simulink model "MMAE_beh_id_and_HighD"  (R2019b)
settings: Solver=FixedStepAuto  StartTime=0.0  StopTime=12  FixedStep=Ts_bp  RelTol=1e-3
values from neighbouring files (symbols this model uses):
  Ts = 0.1    [KinematicBicycleModel.m]    (also in LeftLaneChangeSinusoidalMotionModel.m; LinearizedBicycleModel.m; SimplifiedKinematicBicycleModel.m; amm_rel_test.m)
  Ts_bp = 0.01    [laneChangeSinusoidalFcn.m]    (also in laneChangeSinusoidalJacobianFcn.m; leftLaneChangeParametricFcn.m; leftLaneChangeParametricWithAccFcn.m; leftLaneChangeRelativeFcn.m = 0.1)
  vx = X(2)    [cv_model_fun.m]
  vy = X(4)    [cv_model_fun.m]
  x = X(1)    [KinematicBicycleModel.m]    (also in SimplifiedKinematicBicycleModel.m; behavior_model.m = 0:0.01:20; cca_model_fun.m; ctra_model_fun.m)
  y = X(2)    [KinematicBicycleModel.m]    (also in SimplifiedKinematicBicycleModel.m; behavior_model.m = [distances velocities]; cca_model_fun.m; ctra_model_fun.m)
undefined symbols (not defined in the file or in its folder): ax, P_init, rel_x, sigbuilder_block
libraries: simulink x8, dspswit3 x2, dspstat3 x2
settings Model: Creator=jasprit  LastModifiedBy=jasprit
settings DataIOCC: ReturnWorkspaceOutputs=off
settings DebuggingCC: UnderSpecifiedDimensionMsg=warning  ArithmeticOperatorsInVariantConditions=warning
settings SFSimCC: SimUseLocalCustomCode=off  CustomCodeUndefinedFunction=UseInterfaceOnly
settings RTWCC: RTWUseLocalCustomCode=off

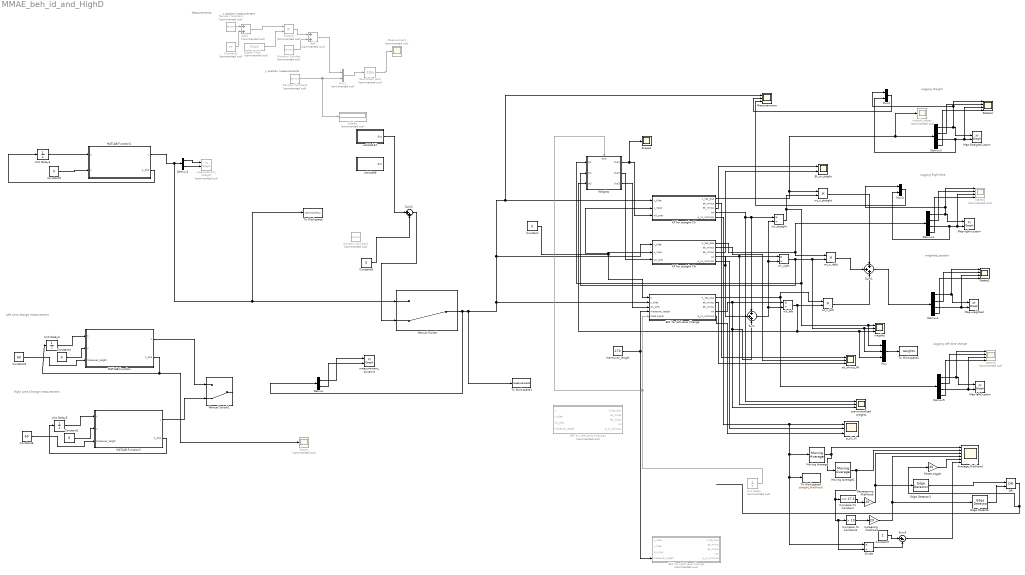
== system MMAE_beh_id_and_HighD ==
  note: Left Lane change measurement
  note: Right Lane Change measurement
  note: Logging Left lane change
  note: Logging straight
  note: Logging Right lane
  note: y position measurements
  note: x position measurement
  note: Measurements
  note: weighted_position
  Add : Sum  Commented=on
  Add1 : Sum  Commented=on
  Average_likelihood : Scope  NumInputPorts=6
  Compare To Constant : simulink/Logic and Bit Operations/Compare To Constant  relop=<=  const=27.5  OutDataTypeStr=boolean
  Compare To Constant1 : simulink/Logic and Bit Operations/Compare To Constant  relop=>  const=10  OutDataTypeStr=boolean
  Constant : Constant  Value=0
  Constant1 : Constant  Value=0  SampleTime=-1
  Constant2 : Constant  Commented=on  Value=vx  SampleTime=Ts
  Constant3 : Constant  Value=60
  Constant4 : Constant  Value=0  SampleTime=-1
  Constant5 : Constant  Value=0  SampleTime=-1
  Constant6 : Constant  Value=60
  Constant7 : Constant
  Constant8 : Constant  Value=0
  Decreasomg likelihood : Gain  Gain=20
  Demux : Demux  Outputs=2
  Demux{1,3..5} (4 alike) : Demux
  Demux2 : Demux  Outputs=2
  Digital Clock : DigitalClock  Commented=on  SampleTime=Ts
  Display : Display  Commented=on
  Divide : Product  Inputs=*/
  EKF for Left Lane Change1 : Subsystem  Commented=on
  EKF for left Lane Change : Subsystem  TreatAsAtomicUnit=on
  EKF for right Lane Change : Subsystem  Commented=on
  Edge Detector : dspswit3/Edge Detector
      settings: SourceProductName=DSP System Toolbox  SourceProductBaseCode=DS
  Edge Detector1 : dspswit3/Edge Detector
      settings: SourceProductName=DSP System Toolbox  SourceProductBaseCode=DS
  Ek_m_stright : Scope  NumInputPorts=2
  Increasing likelihood : Gain  Gain=20
  KF for straight CA : Subsystem
  KF for straight CV : Subsystem
  MATLAB Function : MATLAB Function  TreatAsAtomicUnit=on
  MATLAB Function1 : MATLAB Function  TreatAsAtomicUnit=on
  MATLAB Function2 : MATLAB Function  TreatAsAtomicUnit=on
  Manual Switch : ManualSwitch  CurrentSetting=0
  Manual Switch1 : ManualSwitch  CurrentSetting=0
  Map-StraightCustom : simulink/Sinks/XY Graph  xmin=-1  xmax=200  ymin=-20  ymax=20  st=-1
  Map-leftCustom : simulink/Sinks/XY Graph  xmin=-1  xmax=300  ymin=-5  ymax=5  st=-1
  Map-right-custom : simulink/Sinks/XY Graph  xmin=-1  xmax=300  ymin=-5  ymax=5  st=-1
  Map-weighted : simulink/Sinks/XY Graph  xmin=-1  xmax=300  ymin=-5  ymax=5  st=-1
  "Measurement " : Scope  Commented=on
  Measurements : Scope  NumInputPorts=3
  Moving Average : dspstat3/Moving Average  Method=Sliding window  ForgettingFactorPort=off  SpecifyWindowLength=on  WindowLength=4  ForgettingFactor=0.9  SimulateUsing=Code generation
  Moving Average1 : dspstat3/Moving Average  Method=Sliding window  ForgettingFactorPort=off  SpecifyWindowLength=on  WindowLength=20  ForgettingFactor=0.9  SimulateUsing=Code generation
  Mux : Mux  Inputs=3
  Mux1 : Mux  Commented=on  Inputs=2
  Mux2 : Mux  Inputs=2
  Mux3 : Mux  Inputs=2
  OR : Logic  Operator=OR  IconShape=distinctive  AllPortsSameDT=off  OutDataTypeStr=boolean
  Product : Product  Commented=on
  Random Number : RandomNumber  Commented=on  Variance=0.0025  SampleTime=Ts
  Random Number1 : RandomNumber  Commented=on  Variance=0.0025  SampleTime=Ts
  Random Number2 : RandomNumber  Commented=on  Variance=0.0025  SampleTime=0.01
  Random Number3 : RandomNumber  Commented=on  Variance=0.0025  SampleTime=Ts
  Reset trigger : Gain  Gain=40
  Scope : Scope  Commented=on
  Scope1 : Scope
  States1 : Scope  NumInputPorts=4
  States4 : Scope  NumInputPorts=4
  States5 : Scope  Commented=on  NumInputPorts=4
  States6 : Scope  Commented=on  NumInputPorts=4
  Sum : Sum  Inputs=+++
  Sum1 : Sum  Inputs=+++
  Sum2 : Sum  Inputs=|++
  Sum3 : Sum  Inputs=|+-
  To Workspace : ToWorkspace  VariableName=ground_truth_2  SaveFormat=Timeseries  SampleTime=-1
  To Workspace1 : ToWorkspace  VariableName=measurements  SaveFormat=Timeseries  SampleTime=-1
  To Workspace2 : ToWorkspace  VariableName=weights  SaveFormat=Timeseries  SampleTime=-1
  To Workspace3 : ToWorkspace  VariableName=straight_likelihood  SaveFormat=Timeseries  SampleTime=-1
  Unit Delay : UnitDelay  Commented=on  InitialCondition=[0]  SampleTime=-1  HasFrameUpgradeWarning=on
  Unit Delay3 : UnitDelay  InitialCondition=[x vx y vy]  SampleTime=Ts_bp  HasFrameUpgradeWarning=on
  Unit Delay4 : UnitDelay  InitialCondition=[x vx y vy]  SampleTime=-1  HasFrameUpgradeWarning=on
  Unit Delay5 : UnitDelay  InitialCondition=[x vx y vy]  SampleTime=Ts_bp  HasFrameUpgradeWarning=on
  Weights : Subsystem
  Zero-Order Hold : ZeroOrderHold  Commented=on  SampleTime=Ts
  ek_minus_All : Scope  NumInputPorts=3
  maneuver_length : Constant  Value=270
  measurement_dynamic : simulink/Sinks/XY Graph  xmin=-1  xmax=700  ymin=-5  ymax=20  st=-1
  measurement_straight : simulink/Sinks/XY Graph  Commented=on  xmin=-1  xmax=200  ymin=-5  ymax=5  st=-1
  p_yk_xk : Scope  NumInputPorts=3
  pre-normalized weights : Scope  NumInputPorts=3
  straight_states : Scope  Commented=on
  vehicle167 : Subsystem  Tag=STV Subsys  LoadFcn=sigbuilder_block('load');  StartFcn=sigbuilder_block('start');  StopFcn=sigbuilder_block('stop');  ClipboardFcn=sigbuilder_block('clipboard');  mask(Sigbuilder block){tuvar=[0:10]}
      mask help: Simulink:masks:SigbuilderBlock_MD
      mask init:
      | if ~strcmp(get_param(bdroot(gcbh),'SimulationStatus'),'stopped') tuvar = sigbuilder_block('maskInit'); end
      settings: CopyFcn=sigbuilder_block('copy');  DeleteFcn=sigbuilder_block('delete');  ModelCloseFcn=sigbuilder_block('modelClose');  PreSaveFcn=sigbuilder_block('preSave');  PauseFcn=sigbuilder_block('pause');  ContinueFcn=sigbuilder_block('continue');  NameChangeFcn=sigbuilder_block('namechange');  OpenFcn=sigbuilder_block('open',[437.6 115.5 550.15 399.75 ]);  CloseFcn=sigbuilder_block('close');
      mask Display: plot(0, 0, 100, 100,[2, 2, 32, 32, 2], [68, 8, 8, 68, 68],[32, 2], [38, 38], [32, 19, 2],[53, 60, 44], [32, 17, 17, 2],[16, 16, 31, 31]);txt = getActiveGroup(gcbh);text(2, 100, txt,'verticalAlignment', 'top');
  vehicle99 : Subsystem  Tag=STV Subsys  LoadFcn=sigbuilder_block('load');  StartFcn=sigbuilder_block('start');  StopFcn=sigbuilder_block('stop');  ClipboardFcn=sigbuilder_block('clipboard');  mask(Sigbuilder block){tuvar=[0:10]}
      mask help: Simulink:masks:SigbuilderBlock_MD
      mask init:
      | if ~strcmp(get_param(bdroot(gcbh),'SimulationStatus'),'stopped') tuvar = sigbuilder_block('maskInit'); end
      settings: CopyFcn=sigbuilder_block('copy');  DeleteFcn=sigbuilder_block('delete');  ModelCloseFcn=sigbuilder_block('modelClose');  PreSaveFcn=sigbuilder_block('preSave');  PauseFcn=sigbuilder_block('pause');  ContinueFcn=sigbuilder_block('continue');  NameChangeFcn=sigbuilder_block('namechange');  OpenFcn=sigbuilder_block('open',[2178 24.75 558 422.25 ]);  CloseFcn=sigbuilder_block('close');
      mask Display: plot(0, 0, 100, 100,[2, 2, 32, 32, 2], [68, 8, 8, 68, 68],[32, 2], [38, 38], [32, 19, 2],[53, 60, 44], [32, 17, 17, 2],[16, 16, 31, 31]);txt = getActiveGroup(gcbh);text(2, 100, txt,'verticalAlignment', 'top');
  weights : Scope  NumInputPorts=3
  wk_left : Product  Inputs=*/
  wk_right : Product  Inputs=*/
  wk_straight : Product  Inputs=*/
  wt_x_left : Product  Inputs=**
  wt_x_right : Product  Inputs=**
  wt_x_straight : Product  Inputs=**
  wires:
  Constant2/1 -> Add1/2
  Digital Clock/1 -> Product/2
  Product/1 -> Add/1
  Random Number/1 -> Add/2
  Add/1 -> Mux1/1
  Mux1/1 -> Zero-Order Hold/1
  Random Number3/1 -> Display/1, Mux1/2
  Zero-Order Hold/1 -> "Measurement "/1
  Demux3/1 -> States4/1, Mux2/1, Map-StraightCustom/1
  Demux3/4 -> States4/4
  Demux3/2 -> States4/2
  Demux3/3 -> Mux2/2, Map-StraightCustom/2, States4/3
  Constant/1 -> EKF for left Lane Change/1(u), KF for straight CA/2(u_input), KF for straight CV/2(u_input)
  Demux4/1 -> Mux3/1, States5/1, Map-right-custom/1
  Demux4/2 -> States5/2
  Demux4/4 -> States5/4
  Demux4/3 -> Mux3/2, Map-right-custom/2, States5/3
  Demux5/1 -> States6/1, Map-leftCustom/1
  Demux5/4 -> States6/4
  Demux5/3 -> Map-leftCustom/2, States6/3
  Demux5/2 -> States6/2
  EKF for left Lane Change/1(X_hat_plus) -> wt_x_left/1, Demux5/1
  KF for straight CA/1(X_hat_plus) -> Demux4/1, wt_x_right/1
  KF for straight CV/1(X_hat_plus) -> straight_states/1, Demux3/1, wt_x_straight/1
  EKF for left Lane Change/4(wk) -> wk_left/1, pre-normalized weights/3, Sum/3
  KF for straight CA/4(wk) -> pre-normalized weights/2, wk_right/1, Sum/2
  KF for straight CV/4(wk) -> pre-normalized weights/1, wk_straight/1, Sum/1
  Sum/1 -> wk_left/2, wk_straight/2, wk_right/2
  wk_straight/1 -> Weights/1(In1), Mux/1, weights/1, wt_x_straight/2
  wk_right/1 -> Weights/2(In2), Mux/2, weights/2, wt_x_right/2
  wk_left/1 -> Mux/3, weights/3, Weights/3(In3), wt_x_left/2
  wt_x_right/1 -> Sum1/2
  wt_x_straight/1 -> Sum1/1
  wt_x_left/1 -> Sum1/3
  Demux1/1 -> States1/1, Map-weighted/1
  Demux1/4 -> States1/4
  Demux1/2 -> States1/2
  Demux1/3 -> States1/3, Map-weighted/2
  Sum1/1 -> Demux1/1
  KF for straight CV/2(ek_minus) -> ek_minus_All/1
  KF for straight CA/2(ek_minus) -> ek_minus_All/2
  EKF for left Lane Change/2(ek_minus) -> ek_minus_All/3
  KF for straight CV/5(p_yk_xkminus) -> Moving Average/1, Divide/1, To Workspace3/1, p_yk_xk/1
  KF for straight CA/5(p_yk_xkminus) -> p_yk_xk/2
  EKF for left Lane Change/5(p_yk_xkminus) -> p_yk_xk/3
  KF for straight CV/3(Ek_minus) -> Ek_m_stright/1
  Manual Switch/1 -> To Workspace1/1, KF for straight CA/1(y_tilde), Measurements/1, KF for straight CV/1(y_tilde), EKF for left Lane Change/2(y_tilde), Demux/1
  Unit Delay3/1 -> MATLAB Function/1(X)
  Constant4/1 -> MATLAB Function/2(u)
  Demux/1 -> measurement_dynamic/1
  Demux/2 -> measurement_dynamic/2
  MATLAB Function1/2(X_plus) -> Unit Delay4/1
  Constant5/1 -> MATLAB Function1/2(u)
  Unit Delay4/1 -> MATLAB Function1/1(X)
  MATLAB Function1/1(y) -> To Workspace/1, Manual Switch/1, Demux2/1
  Demux2/1 -> measurement_straight/1
  Demux2/2 -> measurement_straight/2
  MATLAB Function2/2(X_plus) -> Unit Delay5/1
  Unit Delay5/1 -> MATLAB Function2/1(X)
  Constant1/1 -> MATLAB Function2/2(u)
  MATLAB Function/1(y) -> Manual Switch1/1
  MATLAB Function2/1(y) -> Manual Switch1/2
  Random Number1/1 -> Add1/1
  Add1/1 -> Product/1
  maneuver_length/1 -> EKF for left Lane Change/4(maneuver_length), EKF for right Lane Change/4(maneuver_length)
  Constant3/1 -> MATLAB Function/3(maneuver_length)
  Constant6/1 -> MATLAB Function2/3(maneuver_length)
  MATLAB Function/2(X_plus) -> Scope/1, Unit Delay3/1
  Mux/1 -> To Workspace2/1
  Constant8/1 -> Sum2/2
  Sum2/1 -> Manual Switch/2
  Moving Average/1 -> Average_likelihood/1, Moving Average1/1
  Moving Average1/1 -> Divide/2, Compare To Constant1/1, Compare To Constant/1, Average_likelihood/2
  Decreasomg likelihood/1 -> Edge Detector1/1, Average_likelihood/3
  Unit Delay/1 -> Weights/Reset, EKF for left Lane Change/5(reset signal)
  Weights/1(Out1) -> Scope1/1, KF for straight CV/3(wk_prev)
  Weights/2(Out2) -> KF for straight CA/3(wk_prev)
  Weights/3(Out3) -> EKF for left Lane Change/3(wk_prev)
  Compare To Constant/1 -> Decreasomg likelihood/1
  Compare To Constant1/1 -> Increasing likelihood/1
  Increasing likelihood/1 -> Edge Detector/1, Average_likelihood/4
  Edge Detector/1 -> OR/2
  Reset trigger/1 -> Average_likelihood/5
  Edge Detector1/1 -> OR/1
  OR/1 -> Reset trigger/1
  Constant7/1 -> Sum3/1
  Divide/1 -> Sum3/2
  Sum3/1 -> Average_likelihood/6
  KF for straight CA/3(Ek_minus) -> Ek_m_stright/2
  Mux3/1 -> Measurements/3
  Mux2/1 -> Measurements/2
  vehicle167/1(Bus) -> Sum2/1

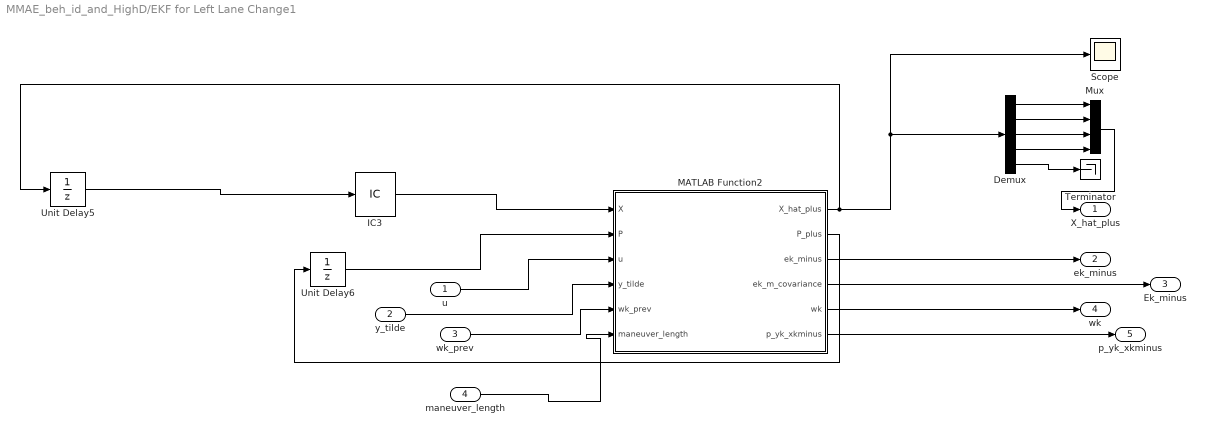
== system MMAE_beh_id_and_HighD/EKF for Left Lane Change1 ==
  u : Inport
  y_tilde : Inport  Port=2
  wk_prev : Inport  Port=3
  maneuver_length : Inport  Port=4
  Demux : Demux  Outputs=5
  IC3 : InitialCondition  Value=[x vx y vy rel_x]
  MATLAB Function2 : MATLAB Function  TreatAsAtomicUnit=on
  Mux : Mux
  Scope : Scope
  Terminator : Terminator
  Unit Delay5 : UnitDelay  SampleTime=-1  HasFrameUpgradeWarning=on
  Unit Delay6 : UnitDelay  InitialCondition=diag([P_init, P_init, P_init, P_init, 200])  SampleTime=-1  HasFrameUpgradeWarning=on
  X_hat_plus : Outport  VectorParamsAs1DForOutWhenUnconnected=off
  ek_minus : Outport  Port=2  VectorParamsAs1DForOutWhenUnconnected=off
  Ek_minus : Outport  Port=3  VectorParamsAs1DForOutWhenUnconnected=off
  wk : Outport  Port=4  VectorParamsAs1DForOutWhenUnconnected=off
  p_yk_xkminus : Outport  Port=5  VectorParamsAs1DForOutWhenUnconnected=off
  wires:
  MATLAB Function2/2(P_plus) -> Unit Delay6/1
  u/1 -> MATLAB Function2/3(u)
  Unit Delay5/1 -> IC3/1
  y_tilde/1 -> MATLAB Function2/4(y_tilde)
  MATLAB Function2/1(X_hat_plus) -> Demux/1, Scope/1, Unit Delay5/1
  IC3/1 -> MATLAB Function2/1(X)
  Unit Delay6/1 -> MATLAB Function2/2(P)
  MATLAB Function2/3(ek_minus) -> ek_minus/1
  MATLAB Function2/4(ek_m_covariance) -> Ek_minus/1
  MATLAB Function2/5(wk) -> wk/1
  MATLAB Function2/6(p_yk_xkminus) -> p_yk_xkminus/1
  wk_prev/1 -> MATLAB Function2/5(wk_prev)
  maneuver_length/1 -> MATLAB Function2/6(maneuver_length)
  Demux/1 -> Mux/1
  Demux/2 -> Mux/2
  Demux/3 -> Mux/3
  Demux/4 -> Mux/4
  Demux/5 -> Terminator/1
  Mux/1 -> X_hat_plus/1

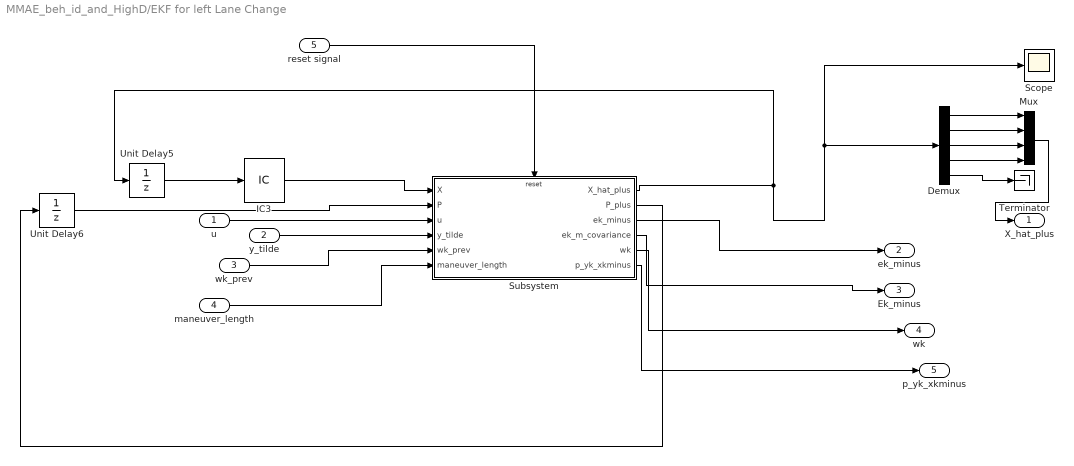
== system MMAE_beh_id_and_HighD/EKF for left Lane Change ==
  u : Inport
  y_tilde : Inport  Port=2
  wk_prev : Inport  Port=3
  maneuver_length : Inport  Port=4
  reset signal : Inport  Port=5
  Demux : Demux  Outputs=5
  IC3 : InitialCondition  Value=[x vx y vy rel_x]
  Mux : Mux
  Scope : Scope
  Subsystem : Subsystem
  Terminator : Terminator
  Unit Delay5 : UnitDelay  InitialCondition=[x vx y vy rel_x]  SampleTime=-1  HasFrameUpgradeWarning=on
  Unit Delay6 : UnitDelay  InitialCondition=diag([P_init, P_init, P_init, P_init, 200])  SampleTime=-1  HasFrameUpgradeWarning=on
  X_hat_plus : Outport  VectorParamsAs1DForOutWhenUnconnected=off
  ek_minus : Outport  Port=2  VectorParamsAs1DForOutWhenUnconnected=off
  Ek_minus : Outport  Port=3  VectorParamsAs1DForOutWhenUnconnected=off
  wk : Outport  Port=4  VectorParamsAs1DForOutWhenUnconnected=off
  p_yk_xkminus : Outport  Port=5  VectorParamsAs1DForOutWhenUnconnected=off
  wires:
  Mux/1 -> X_hat_plus/1
  Demux/4 -> Mux/4
  Demux/5 -> Terminator/1
  Demux/3 -> Mux/3
  Demux/2 -> Mux/2
  Unit Delay5/1 -> IC3/1
  Demux/1 -> Mux/1
  Subsystem/1(X_hat_plus) -> Demux/1, Scope/1, Unit Delay5/1
  IC3/1 -> Subsystem/1(X)
  u/1 -> Subsystem/3(u)
  y_tilde/1 -> Subsystem/4(y_tilde)
  wk_prev/1 -> Subsystem/5(wk_prev)
  maneuver_length/1 -> Subsystem/6(maneuver_length)
  Subsystem/3(ek_minus) -> ek_minus/1
  Subsystem/4(ek_m_covariance) -> Ek_minus/1
  Subsystem/5(wk) -> wk/1
  Subsystem/6(p_yk_xkminus) -> p_yk_xkminus/1
  Unit Delay6/1 -> Subsystem/2(P)
  Subsystem/2(P_plus) -> Unit Delay6/1
  reset signal/1 -> Subsystem/Reset

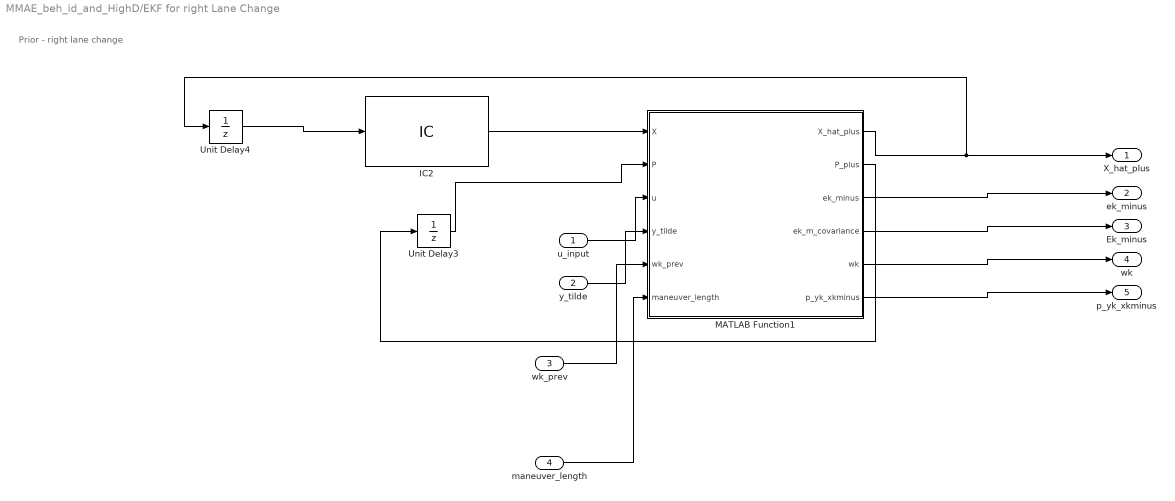
== system MMAE_beh_id_and_HighD/EKF for right Lane Change ==
  note: Prior - right lane change
  u_input : Inport
  y_tilde : Inport  Port=2
  wk_prev : Inport  Port=3
  maneuver_length : Inport  Port=4
  IC2 : InitialCondition  Value=[x vx y vy]
  MATLAB Function1 : MATLAB Function  TreatAsAtomicUnit=on
  Unit Delay3 : UnitDelay  InitialCondition=eye(4)*P_init  SampleTime=-1  HasFrameUpgradeWarning=on
  Unit Delay4 : UnitDelay  SampleTime=-1  HasFrameUpgradeWarning=on
  X_hat_plus : Outport  VectorParamsAs1DForOutWhenUnconnected=off
  ek_minus : Outport  Port=2  VectorParamsAs1DForOutWhenUnconnected=off
  Ek_minus : Outport  Port=3  VectorParamsAs1DForOutWhenUnconnected=off
  wk : Outport  Port=4  VectorParamsAs1DForOutWhenUnconnected=off
  p_yk_xkminus : Outport  Port=5  VectorParamsAs1DForOutWhenUnconnected=off
  wires:
  MATLAB Function1/2(P_plus) -> Unit Delay3/1
  IC2/1 -> MATLAB Function1/1(X)
  Unit Delay3/1 -> MATLAB Function1/2(P)
  MATLAB Function1/1(X_hat_plus) -> X_hat_plus/1, Unit Delay4/1
  u_input/1 -> MATLAB Function1/3(u)
  y_tilde/1 -> MATLAB Function1/4(y_tilde)
  Unit Delay4/1 -> IC2/1
  MATLAB Function1/3(ek_minus) -> ek_minus/1
  MATLAB Function1/4(ek_m_covariance) -> Ek_minus/1
  wk_prev/1 -> MATLAB Function1/5(wk_prev)
  MATLAB Function1/5(wk) -> wk/1
  MATLAB Function1/6(p_yk_xkminus) -> p_yk_xkminus/1
  maneuver_length/1 -> MATLAB Function1/6(maneuver_length)

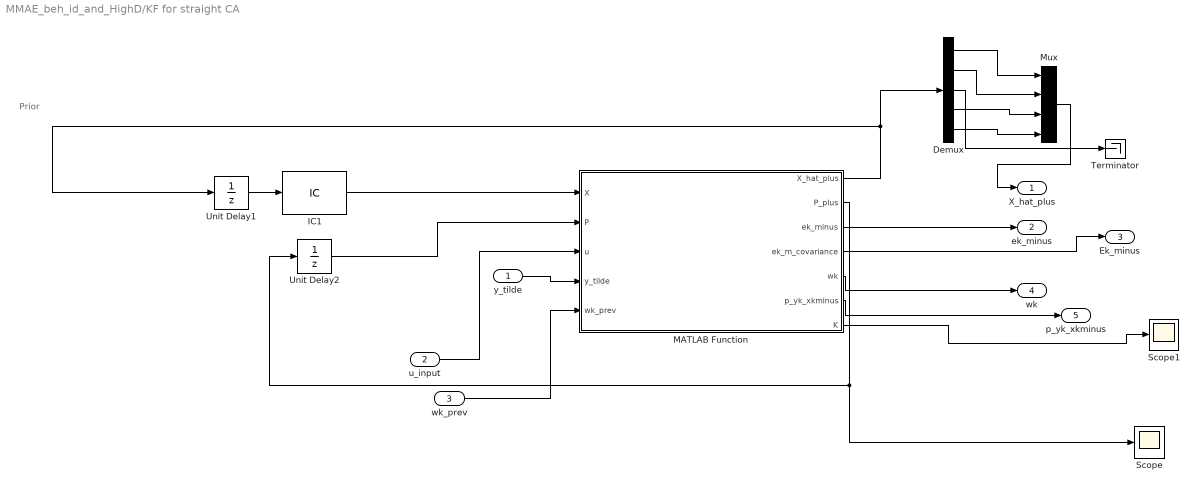
== system MMAE_beh_id_and_HighD/KF for straight CA ==
  note: Prior
  y_tilde : Inport
  u_input : Inport  Port=2
  wk_prev : Inport  Port=3
  Demux : Demux  Outputs=5
  IC1 : InitialCondition  Value=[x vx ax y vy]
  MATLAB Function : MATLAB Function  TreatAsAtomicUnit=on
  Mux : Mux
  Scope : Scope
  Scope1 : Scope
  Terminator : Terminator
  Unit Delay1 : UnitDelay  SampleTime=-1  HasFrameUpgradeWarning=on
  Unit Delay2 : UnitDelay  InitialCondition=eye(5)*P_init  SampleTime=-1  HasFrameUpgradeWarning=on
  X_hat_plus : Outport  VectorParamsAs1DForOutWhenUnconnected=off
  ek_minus : Outport  Port=2  VectorParamsAs1DForOutWhenUnconnected=off
  Ek_minus : Outport  Port=3  VectorParamsAs1DForOutWhenUnconnected=off
  wk : Outport  Port=4  VectorParamsAs1DForOutWhenUnconnected=off
  p_yk_xkminus : Outport  Port=5  VectorParamsAs1DForOutWhenUnconnected=off
  wires:
  Unit Delay2/1 -> MATLAB Function/2(P)
  IC1/1 -> MATLAB Function/1(X)
  MATLAB Function/1(X_hat_plus) -> Demux/1, Unit Delay1/1
  u_input/1 -> MATLAB Function/3(u)
  Unit Delay1/1 -> IC1/1
  y_tilde/1 -> MATLAB Function/4(y_tilde)
  MATLAB Function/2(P_plus) -> Scope/1, Unit Delay2/1
  MATLAB Function/3(ek_minus) -> ek_minus/1
  MATLAB Function/4(ek_m_covariance) -> Ek_minus/1
  wk_prev/1 -> MATLAB Function/5(wk_prev)
  MATLAB Function/5(wk) -> wk/1
  MATLAB Function/6(p_yk_xkminus) -> p_yk_xkminus/1
  MATLAB Function/7(K) -> Scope1/1
  Demux/1 -> Mux/1
  Demux/2 -> Mux/2
  Demux/4 -> Mux/3
  Demux/5 -> Mux/4
  Demux/3 -> Terminator/1
  Mux/1 -> X_hat_plus/1

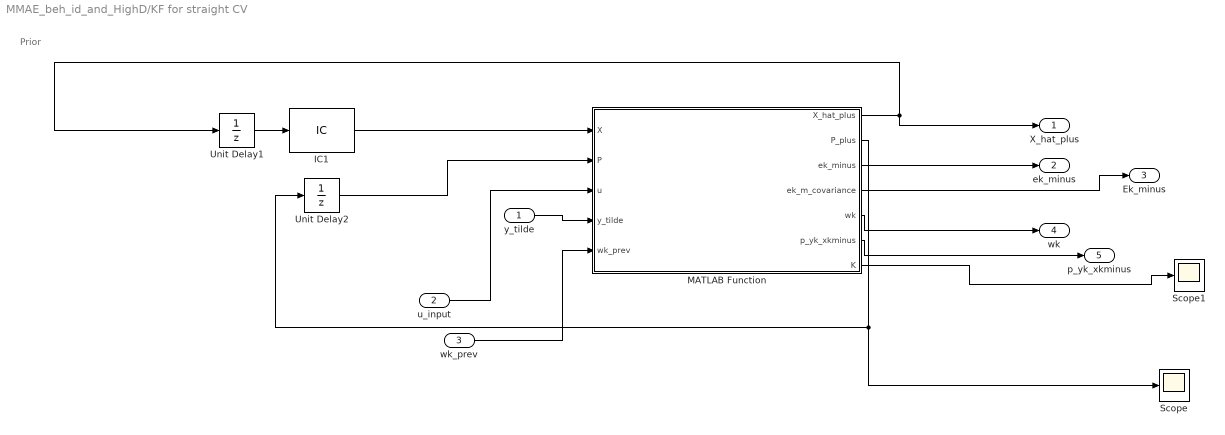
== system MMAE_beh_id_and_HighD/KF for straight CV ==
  note: Prior
  y_tilde : Inport
  u_input : Inport  Port=2
  wk_prev : Inport  Port=3
  IC1 : InitialCondition  Value=[x vx y vy]
  MATLAB Function : MATLAB Function  TreatAsAtomicUnit=on
  Scope : Scope
  Scope1 : Scope
  Unit Delay1 : UnitDelay  SampleTime=-1  HasFrameUpgradeWarning=on
  Unit Delay2 : UnitDelay  InitialCondition=eye(4)*P_init  SampleTime=-1  HasFrameUpgradeWarning=on
  X_hat_plus : Outport  VectorParamsAs1DForOutWhenUnconnected=off
  ek_minus : Outport  Port=2  VectorParamsAs1DForOutWhenUnconnected=off
  Ek_minus : Outport  Port=3  VectorParamsAs1DForOutWhenUnconnected=off
  wk : Outport  Port=4  VectorParamsAs1DForOutWhenUnconnected=off
  p_yk_xkminus : Outport  Port=5  VectorParamsAs1DForOutWhenUnconnected=off
  wires:
  Unit Delay2/1 -> MATLAB Function/2(P)
  IC1/1 -> MATLAB Function/1(X)
  MATLAB Function/1(X_hat_plus) -> X_hat_plus/1, Unit Delay1/1
  u_input/1 -> MATLAB Function/3(u)
  Unit Delay1/1 -> IC1/1
  y_tilde/1 -> MATLAB Function/4(y_tilde)
  MATLAB Function/2(P_plus) -> Scope/1, Unit Delay2/1
  MATLAB Function/3(ek_minus) -> ek_minus/1
  MATLAB Function/4(ek_m_covariance) -> Ek_minus/1
  wk_prev/1 -> MATLAB Function/5(wk_prev)
  MATLAB Function/5(wk) -> wk/1
  MATLAB Function/6(p_yk_xkminus) -> p_yk_xkminus/1
  MATLAB Function/7(K) -> Scope1/1

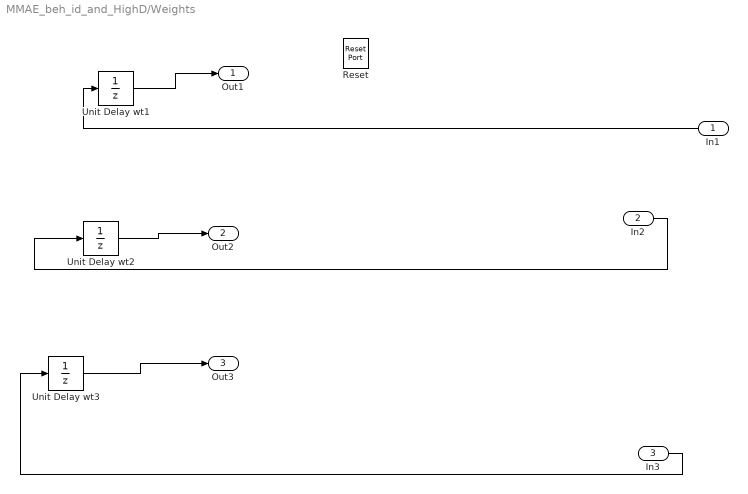
== system MMAE_beh_id_and_HighD/Weights ==
  In1 : Inport
  In2 : Inport  Port=2
  In3 : Inport  Port=3
  Reset : ResetPort  DisableCoverage=on
  Unit Delay wt1 : UnitDelay  InitialCondition=1/3  SampleTime=-1  HasFrameUpgradeWarning=on
  Unit Delay wt2 : UnitDelay  InitialCondition=1/3  SampleTime=-1  HasFrameUpgradeWarning=on
  Unit Delay wt3 : UnitDelay  InitialCondition=1/3  SampleTime=-1  HasFrameUpgradeWarning=on
  Out1 : Outport  VectorParamsAs1DForOutWhenUnconnected=off
  Out2 : Outport  Port=2  VectorParamsAs1DForOutWhenUnconnected=off
  Out3 : Outport  Port=3  VectorParamsAs1DForOutWhenUnconnected=off
  wires:
  In1/1 -> Unit Delay wt1/1
  Unit Delay wt1/1 -> Out1/1
  In2/1 -> Unit Delay wt2/1
  Unit Delay wt2/1 -> Out2/1
  Unit Delay wt3/1 -> Out3/1
  In3/1 -> Unit Delay wt3/1

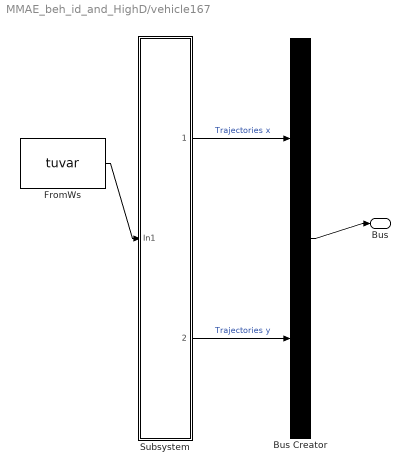
== system MMAE_beh_id_and_HighD/vehicle167 ==
  Bus Creator : BusCreator  Tag=Bus Creator  Inputs=2
  FromWs : FromWorkspace  Tag=STV FromWs  VariableName=tuvar  SampleTime=0
      SigBuilderData=|
      | common.afterFinalStr = 'Extrapolate'
      | common.sampleTime = 0
      | dataSet.timeRange = [0 15]
      | dataSet.name = 'Group 1'
      | sbobj.Groups.Name = 'Group 1'
      | sbobj.Groups.Signals(1).Name = 'Trajectories x'
      | sbobj.Groups.Signals(1).XData = [0 0.04 0.08 0.12 0.16 0.2 0.24 0.28 0.32 0.36 0.4 0.44 0.48 0.52 0.56 0.6 0.64 0.68 0.72 0.76 0.8 0.84 0.88 0.92 0.96 1 1.04 1.08 1.12 1.16 1.2 1.24 1.28 1.32 1.36 1.4 1.44 1.48 1.52 1.56 1.6 1.64 1.68 1.72 1.76 1.8 1.84 1.88 1.92 1.96 2 2.04 2.08 2.12 2.16 2.2 2.24 2.28 2.32 2.36 2.4 2.44 2.48 2.52 2.56 2.6 2.64 2.68 2.72 2.76 2.8 2.84 2.88 2.92 2.96 3 3.04 3.08 3.12 3.16 3.2 3.24 3.28 3.32 3.36 3.4 3.44 3.48 3.52 3.56 3.6 3.64 3.68 3.72 3.76 3.8 3.84 3.88 3.92 3.96 4 4.04 4.08 4.12 4.16 4.2 4.24 4.28 4.32 4.36 4.4 4.44 4.48 4.52 4.56 4.6 4.64 4.68 4.72 4.76 4.8 4.84 4.88 4.92 4.96 5 5.04 5.08 5.12 5.16 5.2 5.24 5.28 5.32 5.36 5.4 5.44 5.48 5.52 5.56 5.6 5.64 5.68 5.72 5.76 5.8 5.84 5.88 5.92 5.96 6 6.04 6.08 6.12 6.16 6.2 6.24 6.28 6.32 6.36 6.4 6.44 6.48 6.52 6.56 6.6 6.64 6.68 6.72 6.76 6.8 6.84 6.88 6.92 6.96 7 7.04 7.08 7.12 7.16 7.2 7.24 7.28 7.32 7.36 7.4 7.44 7.48 7.52 7.56 7.6 7.64 7.68 7.72 7.76 7.8 7.84 7.88 7.92 7.96 8 8.04 8.08 8.12 8.16 8.2 8.24 8.28 8.32 8.36 8.4 8.44 8.48 8.52 8.56 8.6 8.64 8.68 8.72 8.76 8.8 8.84 8.88 8.92 8.96 9 9.04 9.08 9.12 9.16 9.2 9.24 9.28 9.32 9.36 9.4 9.44 9.48 9.52 9.56 9.6 9.64 9.68 9.72 9.76 9.8 9.84 9.88 9.92 9.96 10 10.04 10.08 10.12 10.16 10.2 10.24 10.28 15]
      | sbobj.Groups.Signals(1).YData = [0 1.455632 2.912072 4.369312 5.82736 7.286216 8.74628 10.207152 11.668824 13.131704 14.595392 16.060288 ... (259 elements, 1x259)]
      | sbobj.Groups.Signals(2).Name = 'Trajectories y'
      | sbobj.Groups.Signals(2).XData = [0 0.04 0.08 0.12 0.16 0.2 0.24 0.28 0.32 0.36 0.4 0.44 0.48 0.52 0.56 0.6 0.64 0.68 0.72 0.76 0.8 0.84 0.88 0.92 0.96 1 1.04 1.08 1.12 1.16 1.2 1.24 1.28 1.32 1.36 1.4 1.44 1.48 1.52 1.56 1.6 1.64 1.68 1.72 1.76 1.8 1.84 1.88 1.92 1.96 2 2.04 2.08 2.12 2.16 2.2 2.24 2.28 2.32 2.36 2.4 2.44 2.48 2.52 2.56 2.6 2.64 2.68 2.72 2.76 2.8 2.84 2.88 2.92 2.96 3 3.04 3.08 3.12 3.16 3.2 3.24 3.28 3.32 3.36 3.4 3.44 3.48 3.52 3.56 3.6 3.64 3.68 3.72 3.76 3.8 3.84 3.88 3.92 3.96 4 4.04 4.08 4.12 4.16 4.2 4.24 4.28 4.32 4.36 4.4 4.44 4.48 4.52 4.56 4.6 4.64 4.68 4.72 4.76 4.8 4.84 4.88 4.92 4.96 5 5.04 5.08 5.12 5.16 5.2 5.24 5.28 5.32 5.36 5.4 5.44 5.48 5.52 5.56 5.6 5.64 5.68 5.72 5.76 5.8 5.84 5.88 5.92 5.96 6 6.04 6.08 6.12 6.16 6.2 6.24 6.28 6.32 6.36 6.4 6.44 6.48 6.52 6.56 6.6 6.64 6.68 6.72 6.76 6.8 6.84 6.88 6.92 6.96 7 7.04 7.08 7.12 7.16 7.2 7.24 7.28 7.32 7.36 7.4 7.44 7.48 7.52 7.56 7.6 7.64 7.68 7.72 7.76 7.8 7.84 7.88 7.92 7.96 8 8.04 8.08 8.12 8.16 8.2 8.24 8.28 8.32 8.36 8.4 8.44 8.48 8.52 8.56 8.6 8.64 8.68 8.72 8.76 8.8 8.84 8.88 8.92 8.96 9 9.04 9.08 9.12 9.16 9.2 9.24 9.28 9.32 9.36 9.4 9.44 9.48 9.52 9.56 9.6 9.64 9.68 9.72 9.76 9.8 9.84 9.88 9.92 9.96 10 10.04 10.08 10.12 10.16 10.2 10.24 10.28 15]
      | sbobj.Groups.Signals(2).YData = [0 8e-06 2.4e-05 0.000448 0.00088 0.00132 0.00216 0.003008 0.004264 0.005528 0.007192 0.008864 ... (259 elements, 1x259)]
      | sbobj.Groups.TimeRange = [0 15]
  Subsystem : Subsystem
  Bus : Outport  VectorParamsAs1DForOutWhenUnconnected=off
  wires:
  FromWs/1 -> Subsystem/1(In1)
  Subsystem/1(Trajectories x) -> Bus Creator/1  "Trajectories x"
  Subsystem/2(Trajectories y) -> Bus Creator/2  "Trajectories y"
  Bus Creator/1 -> Bus/1

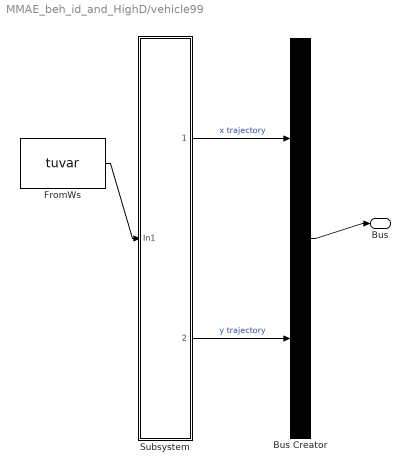
== system MMAE_beh_id_and_HighD/vehicle99 ==
  Bus Creator : BusCreator  Tag=Bus Creator  Inputs=2
  FromWs : FromWorkspace  Tag=STV FromWs  VariableName=tuvar  SampleTime=0
      SigBuilderData=|
      | common.afterFinalStr = 'Extrapolate'
      | common.sampleTime = 0
      | dataSet.timeRange = [0 15]
      | dataSet.name = 'Group 1'
      | sbobj.Groups.Name = 'Group 1'
      | sbobj.Groups.Signals(1).Name = 'x trajectory'
      | sbobj.Groups.Signals(1).XData = [0 0.04 0.08 0.12 0.16 0.2 0.24 0.28 0.32 0.36 0.4 0.44 0.48 0.52 0.56 0.6 0.64 0.68 0.72 0.76 0.8 0.84 0.88 0.92 0.96 1 1.04 1.08 1.12 1.16 1.2 1.24 1.28 1.32 1.36 1.4 1.44 1.48 1.52 1.56 1.6 1.64 1.68 1.72 1.76 1.8 1.84 1.88 1.92 1.96 2 2.04 2.08 2.12 2.16 2.2 2.24 2.28 2.32 2.36 2.4 2.44 2.48 2.52 2.56 2.6 2.64 2.68 2.72 2.76 2.8 2.84 2.88 2.92 2.96 3 3.04 3.08 3.12 3.16 3.2 3.24 3.28 3.32 3.36 3.4 3.44 3.48 3.52 3.56 3.6 3.64 3.68 3.72 3.76 3.8 3.84 3.88 3.92 3.96 4 4.04 4.08 4.12 4.16 4.2 4.24 4.28 4.32 4.36 4.4 4.44 4.48 4.52 4.56 4.6 4.64 4.68 4.72 4.76 4.8 4.84 4.88 4.92 4.96 5 5.04 5.08 5.12 5.16 5.2 5.24 5.28 5.32 5.36 5.4 5.44 5.48 5.52 5.56 5.6 5.64 5.68 5.72 5.76 5.8 5.84 5.88 5.92 5.96 6 6.04 6.08 6.12 6.16 6.2 6.24 6.28 6.32 6.36 6.4 6.44 6.48 6.52 6.56 6.6 6.64 6.68 6.72 6.76 6.8 6.84 6.88 6.92 6.96 7 7.04 7.08 7.12 7.16 7.2 7.24 7.28 7.32 7.36 7.4 7.44 7.48 7.52 7.56 7.6 7.64 7.68 7.72 7.76 7.8 7.84 7.88 7.92 7.96 8 8.04 8.08 8.12 8.16 8.2 8.24 8.28 8.32 8.36 8.4 8.44 8.48 8.52 8.56 8.6 8.64 8.68 8.72 8.76 8.8 8.84 8.88 8.92 8.96 9 9.04 9.08 9.12 9.16 9.2 9.24 9.28 9.32 9.36 9.4 9.44 9.48 9.52 9.56 9.6 9.64 9.68 9.72 9.76 9.8 9.84 9.88 9.92 9.96 10 10.04 10.08 10.12 10.16 10.2 10.24 10.28 10.32 10.36 10.4 10.44 10.48 10.52 10.56 10.6 10.64 10.68 10.72 10.76 10.8 10.84 10.88 10.92 10.96 11 11.04 11.08 11.12 11.16 11.2 11.24 11.28 11.32 11.36 11.4 11.44 11.48 11.52 11.56 11.6 11.64 11.68 11.72 15]
      | sbobj.Groups.Signals(1).YData = [0 1.374552 2.749112 4.124072 5.49944 6.875208 8.251376 9.627544 11.00412 12.381096 13.758472 15.136248 ... (295 elements, 1x295)]
      | sbobj.Groups.Signals(2).Name = 'y trajectory'
      | sbobj.Groups.Signals(2).XData = [0 0.04 0.08 0.12 0.16 0.2 0.24 0.28 0.32 0.36 0.4 0.44 0.48 0.52 0.56 0.6 0.64 0.68 0.72 0.76 0.8 0.84 0.88 0.92 0.96 1 1.04 1.08 1.12 1.16 1.2 1.24 1.28 1.32 1.36 1.4 1.44 1.48 1.52 1.56 1.6 1.64 1.68 1.72 1.76 1.8 1.84 1.88 1.92 1.96 2 2.04 2.08 2.12 2.16 2.2 2.24 2.28 2.32 2.36 2.4 2.44 2.48 2.52 2.56 2.6 2.64 2.68 2.72 2.76 2.8 2.84 2.88 2.92 2.96 3 3.04 3.08 3.12 3.16 3.2 3.24 3.28 3.32 3.36 3.4 3.44 3.48 3.52 3.56 3.6 3.64 3.68 3.72 3.76 3.8 3.84 3.88 3.92 3.96 4 4.04 4.08 4.12 4.16 4.2 4.24 4.28 4.32 4.36 4.4 4.44 4.48 4.52 4.56 4.6 4.64 4.68 4.72 4.76 4.8 4.84 4.88 4.92 4.96 5 5.04 5.08 5.12 5.16 5.2 5.24 5.28 5.32 5.36 5.4 5.44 5.48 5.52 5.56 5.6 5.64 5.68 5.72 5.76 5.8 5.84 5.88 5.92 5.96 6 6.04 6.08 6.12 6.16 6.2 6.24 6.28 6.32 6.36 6.4 6.44 6.48 6.52 6.56 6.6 6.64 6.68 6.72 6.76 6.8 6.84 6.88 6.92 6.96 7 7.04 7.08 7.12 7.16 7.2 7.24 7.28 7.32 7.36 7.4 7.44 7.48 7.52 7.56 7.6 7.64 7.68 7.72 7.76 7.8 7.84 7.88 7.92 7.96 8 8.04 8.08 8.12 8.16 8.2 8.24 8.28 8.32 8.36 8.4 8.44 8.48 8.52 8.56 8.6 8.64 8.68 8.72 8.76 8.8 8.84 8.88 8.92 8.96 9 9.04 9.08 9.12 9.16 9.2 9.24 9.28 9.32 9.36 9.4 9.44 9.48 9.52 9.56 9.6 9.64 9.68 9.72 9.76 9.8 9.84 9.88 9.92 9.96 10 10.04 10.08 10.12 10.16 10.2 10.24 10.28 10.32 10.36 10.4 10.44 10.48 10.52 10.56 10.6 10.64 10.68 10.72 10.76 10.8 10.84 10.88 10.92 10.96 11 11.04 11.08 11.12 11.16 11.2 11.24 11.28 11.32 11.36 11.4 11.44 11.48 11.52 11.56 11.6 11.64 11.68 11.72 11.72 15]
      | sbobj.Groups.Signals(2).YData = [0 0 0.000408 0.000816 0.001224 0.001632 0.00244 0.003248 0.004056 0.004872 0.006088 0.007304 ... (296 elements, 1x296)]
      | sbobj.Groups.TimeRange = [0 15]
  Subsystem : Subsystem
  Bus : Outport  VectorParamsAs1DForOutWhenUnconnected=off
  wires:
  FromWs/1 -> Subsystem/1(In1)
  Subsystem/1(x trajectory) -> Bus Creator/1  "x trajectory"
  Subsystem/2(y trajectory) -> Bus Creator/2  "y trajectory"
  Bus Creator/1 -> Bus/1

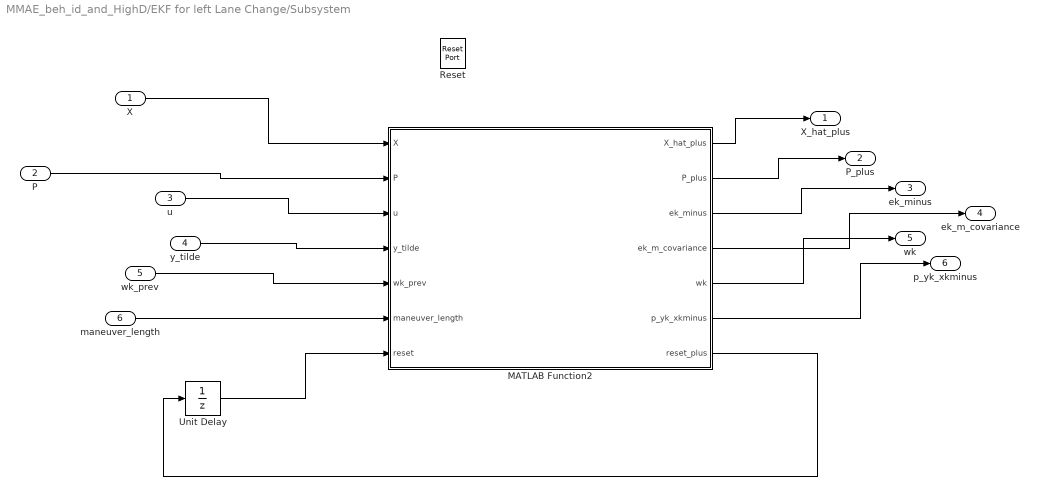
== system MMAE_beh_id_and_HighD/EKF for left Lane Change/Subsystem ==
  X : Inport
  P : Inport  Port=2
  u : Inport  Port=3
  y_tilde : Inport  Port=4
  wk_prev : Inport  Port=5
  maneuver_length : Inport  Port=6
  Reset : ResetPort  DisableCoverage=on
  MATLAB Function2 : MATLAB Function  TreatAsAtomicUnit=on
  Unit Delay : UnitDelay  SampleTime=-1  HasFrameUpgradeWarning=on
  X_hat_plus : Outport  VectorParamsAs1DForOutWhenUnconnected=off
  P_plus : Outport  Port=2  VectorParamsAs1DForOutWhenUnconnected=off
  ek_minus : Outport  Port=3  VectorParamsAs1DForOutWhenUnconnected=off
  ek_m_covariance : Outport  Port=4  VectorParamsAs1DForOutWhenUnconnected=off
  wk : Outport  Port=5  VectorParamsAs1DForOutWhenUnconnected=off
  p_yk_xkminus : Outport  Port=6  VectorParamsAs1DForOutWhenUnconnected=off
  wires:
  MATLAB Function2/5(wk) -> wk/1
  MATLAB Function2/1(X_hat_plus) -> X_hat_plus/1
  X/1 -> MATLAB Function2/1(X)
  P/1 -> MATLAB Function2/2(P)
  u/1 -> MATLAB Function2/3(u)
  wk_prev/1 -> MATLAB Function2/5(wk_prev)
  MATLAB Function2/3(ek_minus) -> ek_minus/1
  y_tilde/1 -> MATLAB Function2/4(y_tilde)
  maneuver_length/1 -> MATLAB Function2/6(maneuver_length)
  MATLAB Function2/2(P_plus) -> P_plus/1
  MATLAB Function2/6(p_yk_xkminus) -> p_yk_xkminus/1
  MATLAB Function2/4(ek_m_covariance) -> ek_m_covariance/1
  Unit Delay/1 -> MATLAB Function2/7(reset)
  MATLAB Function2/7(reset_plus) -> Unit Delay/1

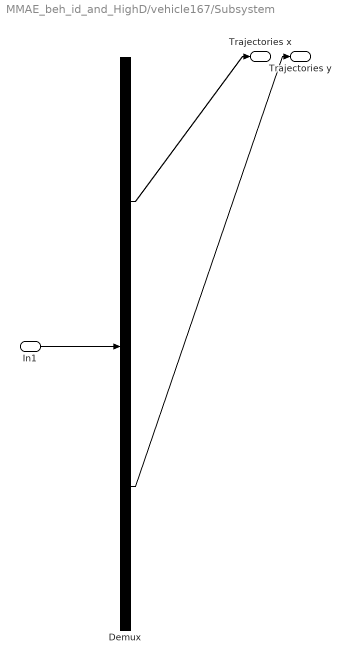
== system MMAE_beh_id_and_HighD/vehicle167/Subsystem ==
  In1 : Inport
  Demux : Demux  Tag=STV Demux  Outputs=2
  Trajectories x : Outport  Tag=STV Outport  VectorParamsAs1DForOutWhenUnconnected=off
  Trajectories y : Outport  Tag=STV Outport  Port=2  VectorParamsAs1DForOutWhenUnconnected=off
  wires:
  Demux/1 -> Trajectories x/1
  Demux/2 -> Trajectories y/1
  In1/1 -> Demux/1

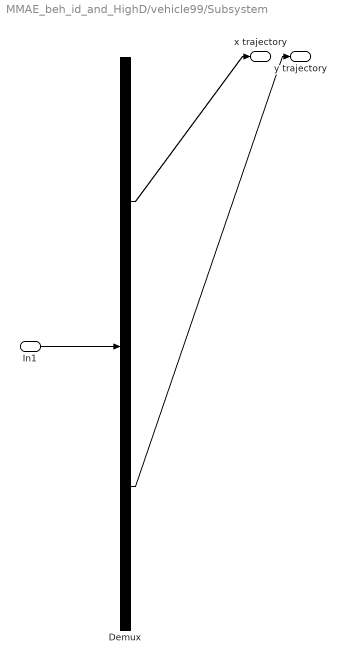
== system MMAE_beh_id_and_HighD/vehicle99/Subsystem ==
  In1 : Inport
  Demux : Demux  Tag=STV Demux  Outputs=2
  x trajectory : Outport  Tag=STV Outport  VectorParamsAs1DForOutWhenUnconnected=off
  y trajectory : Outport  Tag=STV Outport  Port=2  VectorParamsAs1DForOutWhenUnconnected=off
  wires:
  Demux/1 -> x trajectory/1
  Demux/2 -> y trajectory/1
  In1/1 -> Demux/1

== matlab function MMAE_beh_id_and_HighD/EKF for right Lane Change/MATLAB Function1 ==
  data: X input; P input; u input; X_hat_plus output; y_tilde input; P_plus output; ek_minus output; ek_m_covariance output; wk output; p_yk_xkminus output; wk_prev input; maneuver_length input
function [X_hat_plus, P_plus, ek_minus, ek_m_covariance, wk, p_yk_xkminus] = EKFRightLaneChangeCustom(X, P, u, y_tilde, wk_prev, maneuver_length)

    %%
    %TODO: See how can this be moved out of the function later
    %sampling time
    Ts_bp = 0.1;
%     maneuver_length = 150;  %m
    lane_center_to_center_distance = 3.5;   %meters

    % measurement noise covariance
%      R = [0.25 0; 0 0.25];
   R = [0.0025 0; 0 0.0025];
    
    % process noise covariance
%     Q = diag([0.5 5.0 0.5 5.0]);
%     Q = diag([0.001 0.01 0.001 0.01]);
    Q = diag([0.05 0.01 0.05 0.01]);

    % states - X = [x vx y vy] -     
    Ck = [1 0 0 0; 0 0 1 0];

    F = rightLaneChangeParametricJacobianFcn(X, u, maneuver_length, lane_center_to_center_distance);
    %%
    % Now estimate states using kalman filter
    
    %predict
    xhat_minus = rightLaneChangeParametricFcn(X, u, maneuver_length, lane_center_to_center_distance);
    P_minus = (F * P * F') + Ts_bp*Q;
    yhat_minus = Ck * xhat_minus;

    %correct
    ek_minus = y_tilde - yhat_minus;    %residual
    ek_m_covariance = Ck * P_minus *Ck' + R;    %residual covariance
    K = P_minus * Ck' * inv(ek_m_covariance);
    X_hat_plus = xhat_minus + K * ek_minus;
    P_plus = (eye(4) - K * Ck) * P_minus;

    %calculate MMAE weights
    p_yk_xkminus = 1/sqrt(det(2*pi*ek_m_covariance))*exp(-1/2 * ek_minus'* inv(ek_m_covariance) * ek_minus);
    wk = wk_prev * p_yk_xkminus;

end

== matlab function MMAE_beh_id_and_HighD/KF for straight CV/MATLAB Function ==
  data: X input; P input; u input; X_hat_plus output; y_tilde input; P_plus output; ek_minus output; ek_m_covariance output; wk output; wk_prev input; p_yk_xkminus output; K output
function [X_hat_plus, P_plus, ek_minus, ek_m_covariance, wk, p_yk_xkminus, K] = kalmanFilterCustom(X, P, u, y_tilde, wk_prev)

    %%
    %TODO: See how can this be moved out of the function later
    %sampling time
    Ts_bp = 0.1;

    % measurement noise covariance
%      R = [0.25 0; 0 0.25];
   R = [0.0025 0; 0 0.0025];
    
    % process noise covariance
%     Q = diag([0.5 5.0 0.5 5.0]);
%     Q = diag([0.001 0.01 0.001 0.01]);
%     Q = diag([0.01 0.01 0.05 0.01]);
    % acceleration noise = 0.85 m/s2 std dev, variance = 0.7225
    a = Ts_bp^4/4;
    b = Ts_bp^3/2;
    c = Ts_bp^2;
    std_dev_q = 0.85; %m/s2
    var_q = 0.7225; %std_dev_q^2
    Q = var_q * [a b 0 0; b c 0 0; 0 0 a b; 0 0 b c];
%      Q = var_q * [0.01 0 0 0; 0 0.01 0 0; 0 0 var_q*a 0; 0 0 0 var_q*c];

    % states - X = [x vx y vy] - 
    
%     Ak = [1 Ts_bp 0 0; 0 1 0 0; 0 0 1 Ts_bp; 0 0 0 1];
    Ak = [1 Ts_bp 0 0; 0 1 0 0; 0 0 1 0; 0 0 0 0];
    Bk = 0;
    Ck = [1 0 0 0; 0 0 1 0];
    Dk = 0;

    %%
    % Now estimate states using kalman filter
    
    %predict
    xhat_minus = Ak * X + Bk * u;
%     P_minus = (Ak * P *Ak') + Ts_bp*Q;
    P_minus = (Ak * P *Ak') + Q;
    yhat_minus = Ck * xhat_minus;

    %correct
    ek_minus = y_tilde - yhat_minus;    %residual
    ek_m_covariance = Ck * P_minus *Ck' + R;    %residual covariance
    K = P_minus * Ck' * inv(ek_m_covariance);
    X_hat_plus = xhat_minus + K * ek_minus;
    P_plus = (eye(4) - K * Ck) * P_minus;
    
    %calculate MMAE weights
%     p_yk_xkminus = 1/sqrt(det(2*pi*ek_m_covariance))*exp(-1/2 * ek_minus'* inv(ek_m_covariance) * ek_minus);
    p_yk_xkminus = 1/sqrt(det((2*pi)^2*ek_m_covariance))*exp(-1/2 * ek_minus'* inv(ek_m_covariance) * ek_minus);
%     p_yk_xkminus = 1/sqrt(det((2*pi)*ek_m_covariance(2,2)))*exp(-1/2 * ek_minus(2)^2* inv(ek_m_covariance(2,2)));
    wk = wk_prev * p_yk_xkminus;
    
    %This will be likely outside
    %e = xhat_plus - x(:, i+1);
    
end

== matlab function MMAE_beh_id_and_HighD/EKF for left Lane Change/Subsystem/MATLAB Function2 ==
  data: X input; P input; u input; X_hat_plus output; y_tilde input; P_plus output; ek_minus output; ek_m_covariance output; wk output; p_yk_xkminus output; wk_prev input; maneuver_length input; reset input; reset_plus output
function [X_hat_plus, P_plus, ek_minus, ek_m_covariance, wk, p_yk_xkminus, reset_plus] = EKFLeftLaneChangeCustom(X, P, u, y_tilde, wk_prev, maneuver_length, reset)

    %%
    %TODO: See how can this be moved out of the function later
    %sampling time    
    Ts_bp = 0.1;
    
    persistent motionModel;
    
    if isempty(motionModel)
        lane_center_to_center_distance = 3.5;   %meters, usually the lane width
        motionModel = LeftLaneChangeRelativeMotionModel(Ts_bp, maneuver_length, lane_center_to_center_distance);
    end

    % measurement noise covariance
%      R = [0.25 0; 0 0.25];
   R = [0.0025 0; 0 0.0025];
    
    % process noise covariance
%     Q = diag([0.5 5.0 0.5 5.0]);
%    Q = diag([0.001 0.001 0.001 0.001 0.001]);
%     Q = diag([0.001 0.01 0.001 0.01]);
    Q = diag([0.5 0.01 0.5 0.01 0.001]);

    % states - X = [x vx y vy x0] -     
    Ck = [1 0 0 0 0 ; 0 0 1 0 0];

    if reset == 1
        reset = 0;
        
        % x0 = x, update the initiation point to x and reset the covariance
        X(5) = X(1);
        P(5,5) = 50;
    end
    
    reset_plus = reset;
    
%     F = leftLaneChangeRelativeJacobianFcn(X, u, maneuver_length, lane_center_to_center_distance);
    F = motionModel.jacobian_propagation(X, u);
    %%
    % Now estimate states using kalman filter
    
    %predict
%     xhat_minus = leftLaneChangeRelativeFcn(X, u, maneuver_length, lane_center_to_center_distance);
    xhat_minus =  motionModel.propagate(X, u);
    P_minus = (F * P * F') + Ts_bp*Q;
    yhat_minus = Ck * xhat_minus;

    %correct
    ek_minus = y_tilde - yhat_minus;    %residual
    ek_m_covariance = Ck * P_minus *Ck' + R;    %residual covariance
    K = P_minus * Ck' * inv(ek_m_covariance);
    X_hat_plus = xhat_minus + K * ek_minus;
    P_plus = (eye(5) - K * Ck) * P_minus;
    
    %calculate MMAE weights
 %     p_yk_xkminus = 1/sqrt(det(2*pi*ek_m_covariance))*exp(-1/2 * ek_minus'* inv(ek_m_covariance) * ek_minus);
    p_yk_xkminus = 1/sqrt(det((2*pi)^2*ek_m_covariance))*exp(-1/2 * ek_minus'* inv(ek_m_covariance) * ek_minus);
   wk = wk_prev * p_yk_xkminus;
    
end

== matlab function MMAE_beh_id_and_HighD/MATLAB Function ==
  data: X input; u input; y output; X_plus output; maneuver_length input
function [y, X_plus]= measurementsForLaneChange(X, u, maneuver_length)

    Ts_bp = 0.01;
%     maneuver_length = 150;  %m
    lane_center_to_center_distance = 3.5;   %meters

    % states - X = [x vx y vy] -     
    Ck = [1 0 0 0; 0 0 1 0];

    % measurement noise std_dev
%     R_sigma = [0.5 0; 0 0.5];
   R_sigma = [0.05 0; 0 0.05];
    
    % process noise std dev
%    sigma_matrix = diag([0.16 0.16 0.16 0.16]);
    sigma_matrix = diag([0.032 0.032 0.032 0.032]);
    
%     if t < 15
%         Ak = [1 Ts 0 0; 0 1 0 0; 0 0 1 Ts; 0 0 0 1];
%         Bk = 0;
%         X_plus = Ak * X + Bk * u + sqrt(Ts) * sigma_matrix * randn(4,1);
%     else
        X_plus = leftLaneChangeParametricFcn(X, u, maneuver_length, lane_center_to_center_distance) + sqrt(Ts_bp)*sigma_matrix*randn(4,1);    
%     end
    
    y = Ck * X_plus + R_sigma * randn(2,1);
    
end

== matlab function MMAE_beh_id_and_HighD/MATLAB Function1 ==
  data: X input; u input; y output; X_plus output
function [y, X_plus]= measurementsForStraightMotion(X, u)

    Ts_bp = 0.01;
    % states - X = [x vx y vy] -     
    Ak = [1 Ts_bp 0 0; 0 1 0 0; 0 0 1 Ts_bp; 0 0 0 1];
    Bk = 0;
    Ck = [1 0 0 0; 0 0 1 0];

    % measurement noise std_dev
%     R_sigma = [0.5 0; 0 0.5];
   R_sigma = [0.05 0; 0 0.05];
    
    % process noise std dev
%    sigma_matrix = diag([0.16 0.16 0.16 0.16]);
    sigma_matrix = diag([0.032 0.032 0.032 0.032]);
  
    X(3) = 0;
%    X(4) = 0;
    
    X_plus = Ak * X + Bk * u + sqrt(Ts_bp)*sigma_matrix*randn(4,1);    
    
    y = Ck * X_plus + R_sigma * randn(2,1);
    
end

== matlab function MMAE_beh_id_and_HighD/MATLAB Function2 ==
  data: X input; u input; y output; X_plus output; maneuver_length input
function [y, X_plus]= measurementsForLaneChange(X, u, maneuver_length)

    Ts_bp = 0.01;
%    maneuver_length = 150;  %m
    lane_center_to_center_distance = 3.5;   %meters

    % states - X = [x vx y vy] -     
    Ck = [1 0 0 0; 0 0 1 0];

    % measurement noise std_dev
%     R_sigma = [0.5 0; 0 0.5];
   R_sigma = [0.05 0; 0 0.05];
    
    % process noise std dev
%    sigma_matrix = diag([0.16 0.16 0.16 0.16]);
    sigma_matrix = diag([0.032 0.032 0.032 0.032]);
    
%     if t < 15
%         Ak = [1 Ts 0 0; 0 1 0 0; 0 0 1 Ts; 0 0 0 1];
%         Bk = 0;
%         X_plus = Ak * X + Bk * u + sqrt(Ts) * sigma_matrix * randn(4,1);
%     else
        X_plus = rightLaneChangeParametricFcn(X, u, maneuver_length, lane_center_to_center_distance) + sqrt(Ts_bp)*sigma_matrix*randn(4,1);    
%     end
    
    y = Ck * X_plus + R_sigma * randn(2,1);
    
end

== matlab function MMAE_beh_id_and_HighD/EKF for Left Lane Change1/MATLAB Function2 ==
  data: X input; P input; u input; X_hat_plus output; y_tilde input; P_plus output; ek_minus output; ek_m_covariance output; wk output; p_yk_xkminus output; wk_prev input; maneuver_length input
function [X_hat_plus, P_plus, ek_minus, ek_m_covariance, wk, p_yk_xkminus] = EKFLeftLaneChangeCustom(X, P, u, y_tilde, wk_prev, maneuver_length)

    %%
    %TODO: See how can this be moved out of the function later
    %sampling time
    Ts_bp = 0.01;
%     maneuver_length = 150;  %m
    lane_center_to_center_distance = 3.5;   %meters

    % measurement noise covariance
%      R = [0.25 0; 0 0.25];
   R = [0.0025 0; 0 0.0025];
    
    % process noise covariance
%     Q = diag([0.5 5.0 0.5 5.0]);
    Q = diag([0.001 0.001 0.001 0.001 0.001]);

    % states - X = [x vx y vy] -     
    Ck = [1 0 0 0 0 ; 0 0 1 0 0];

    F = leftLaneChangeRelativeJacobianFcn(X, u, maneuver_length, lane_center_to_center_distance);
    %%
    % Now estimate states using kalman filter
    
    %predict
    xhat_minus = leftLaneChangeRelativeFcn(X, u, maneuver_length, lane_center_to_center_distance);
    P_minus = (F * P * F') + Ts_bp*Q;
    yhat_minus = Ck * xhat_minus;

    %correct
    ek_minus = y_tilde - yhat_minus;    %residual
    ek_m_covariance = Ck * P_minus *Ck' + R;    %residual covariance
    K = P_minus * Ck' * inv(ek_m_covariance);
    X_hat_plus = xhat_minus + K * ek_minus;
    P_plus = (eye(5) - K * Ck) * P_minus;
    
    %calculate MMAE weights
    p_yk_xkminus = 1/sqrt(det(2*pi*ek_m_covariance))*exp(-1/2 * ek_minus'* inv(ek_m_covariance) * ek_minus);
    wk = wk_prev * p_yk_xkminus;

    
end

== matlab function MMAE_beh_id_and_HighD/KF for straight CA/MATLAB Function ==
  data: X input; P input; u input; X_hat_plus output; y_tilde input; P_plus output; ek_minus output; ek_m_covariance output; wk output; wk_prev input; p_yk_xkminus output; K output
function [X_hat_plus, P_plus, ek_minus, ek_m_covariance, wk, p_yk_xkminus, K] = kalmanFilterCustom(X, P, u, y_tilde, wk_prev)

    %%
    %TODO: See how can this be moved out of the function later
    %sampling time
    Ts_bp = 0.1;

    % measurement noise covariance
%      R = [0.25 0; 0 0.25];
   R = [0.0025 0; 0 0.0025];
    
    % process noise covariance
%     Q = diag([0.5 5.0 0.5 5.0]);
%     Q = diag([0.001 0.01 0.001 0.01]);
%    Q = diag([0.01 .01 0.5 0.05 0.01]);
    a = Ts_bp^4/4;
    b = Ts_bp^3/2;
    c = Ts_bp^2;
    std_dev_q = 0.85; %m/s2
    var_q = 0.7225; %std_dev_q^2
    Q = var_q * [a b c/2 0 0; b c Ts_bp 0 0; c/2 Ts_bp 1 0 0; 0 0 0 a b; 0 0 0 b c];
%      Q = var_q * [0.01 0 0 0 0; 0 0.01 0 0 0; 0 0 0.5 0 0; 0 0 0 var_q*a 0; 0 0 0 0 var_q*c];


    % states - X = [x vx y vy] - 
    
%     Ak = [1 Ts_bp 0 0; 0 1 0 0; 0 0 1 Ts_bp; 0 0 0 1];
    Ak = [1 Ts_bp Ts_bp^2/2 0 0; 0 1 Ts_bp 0 0; 0 0 1 0 0; 0 0 0 1 Ts_bp; 0 0 0 0 0];
    Bk = 0;
    Ck = [1 0 0 0 0; 0 0 0 1 0];
    Dk = 0;

    %%
    % Now estimate states using kalman filter
    
    %predict
    xhat_minus = Ak * X + Bk * u;
%     P_minus = (Ak * P *Ak') + Ts_bp*Q;
    P_minus = (Ak * P *Ak') + Q;
    yhat_minus = Ck * xhat_minus;

    %correct
    ek_minus = y_tilde - yhat_minus;    %residual
    ek_m_covariance = Ck * P_minus *Ck' + R;    %residual covariance
    K = P_minus * Ck' * inv(ek_m_covariance);
    X_hat_plus = xhat_minus + K * ek_minus;
    P_plus = (eye(5) - K * Ck) * P_minus;
    
    %calculate MMAE weights
%     p_yk_xkminus = 1/sqrt(det(2*pi*ek_m_covariance))*exp(-1/2 * ek_minus'* inv(ek_m_covariance) * ek_minus);
    p_yk_xkminus = 1/sqrt(det((2*pi)^2*ek_m_covariance))*exp(-1/2 * ek_minus'* inv(ek_m_covariance) * ek_minus);
%     p_yk_xkminus = 1/sqrt(det((2*pi)*ek_m_covariance(2,2)))*exp(-1/2 * ek_minus(2)^2* inv(ek_m_covariance(2,2)));
    wk = wk_prev * p_yk_xkminus;
    
    %This will be likely outside
    %e = xhat_plus - x(:, i+1);
    
end
